simulink model "V605_PropTables"  (R2025a)
settings: Solver=VariableStepAuto  StartTime=0.0  StopTime=10.0  RelTol=1e-3
undefined symbols (not defined in the file or in its folder): prop, rad, s
libraries: aerolibconvert2 x1
settings Model: Creator=Ayush_S  LastModifiedBy=Ayush_S

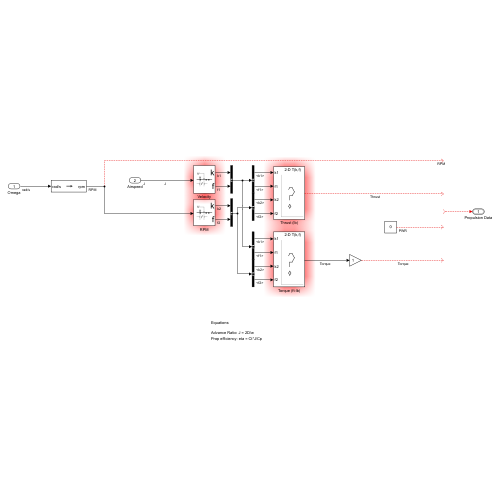
[thumbnail: Simulink's stored preview of the top-level diagram]
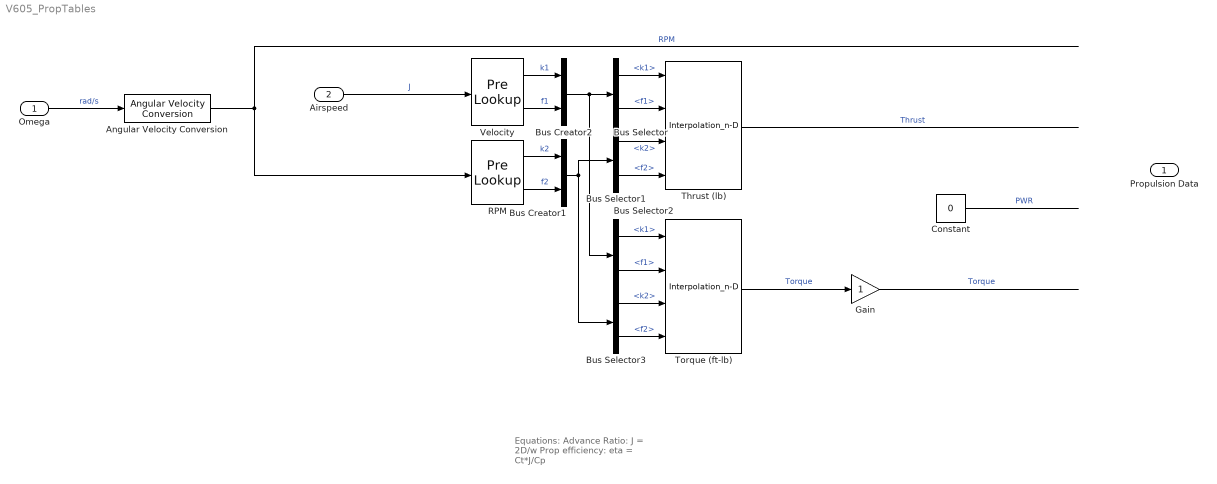
== system V605_PropTables ==
  note: Equations:
      |
      | Advance Ratio: J = 2D/w
      | Prop efficiency: eta = Ct*J/Cp
  Omega : Inport
  Airspeed : Inport  Port=2
  Angular Velocity Conversion : aerolibconvert2/Angular Velocity Conversion  IU=rad/s  OU=rpm
  Bus Creator1 : BusCreator  Inputs=2
  Bus Creator2 : BusCreator  Inputs=2
  Bus Selector : BusSelector  OutputSignals=k1,f1
  Bus Selector1 : BusSelector  OutputSignals=k2,f2
  Bus Selector2 : BusSelector  OutputSignals=k1,f1
  Bus Selector3 : BusSelector  OutputSignals=k2,f2
  Constant : Constant  Value=0
  Gain : Gain
  RPM : PreLookup  BreakpointsData=prop.RPM  ExtrapMethod=Linear
  Thrust (lb) : Interpolation_n-D  Table=prop.Thrust  InternalRulePriority=Speed
  Torque (ft-lb) : Interpolation_n-D  Table=prop.Torque  ExtrapMethod=Clip  InternalRulePriority=Speed
  Velocity : PreLookup  BreakpointsData=prop.vel
  Propulsion Data : Outport  OutDataTypeStr=Bus: PropulsionBus
  wires:
  Velocity/1 -> Bus Creator2/1  "k1"
  Omega/1 -> Angular Velocity Conversion/1  "rad/s"
  Bus Selector3/1 -> Torque (ft-lb)/3  "<k2>"
  Bus Selector1/1 -> Thrust (lb)/3  "<k2>"
  Constant/1 -> ?  "PWR"
  Gain/1 -> ?  "Torque"
  RPM/2 -> Bus Creator1/2  "f2"
  Thrust (lb)/1 -> ?  "Thrust"
  Bus Selector/2 -> Thrust (lb)/2  "<f1>"
  Bus Selector2/1 -> Torque (ft-lb)/1  "<k1>"
  RPM/1 -> Bus Creator1/1  "k2"
  Bus Selector2/2 -> Torque (ft-lb)/2  "<f1>"
  Torque (ft-lb)/1 -> Gain/1  "Torque"
  Bus Selector1/2 -> Thrust (lb)/4  "<f2>"
  Angular Velocity Conversion/1 -> RPM/1  "RPM"
  ? -> Propulsion Data/1
  Bus Creator1/1 -> Bus Selector1/1, Bus Selector3/1
  Bus Selector3/2 -> Torque (ft-lb)/4  "<f2>"
  Bus Creator2/1 -> Bus Selector/1, Bus Selector2/1
  Airspeed/1 -> Velocity/1  "J"
  Velocity/2 -> Bus Creator2/2  "f1"
  Bus Selector/1 -> Thrust (lb)/1  "<k1>"
